simulink model "Exer2"  (R2014b)
settings: Solver=ode45  StartTime=0.0  StopTime=2  RelTol=1e-3
settings Model: Creator=Charlie  LastModifiedBy=Charlie

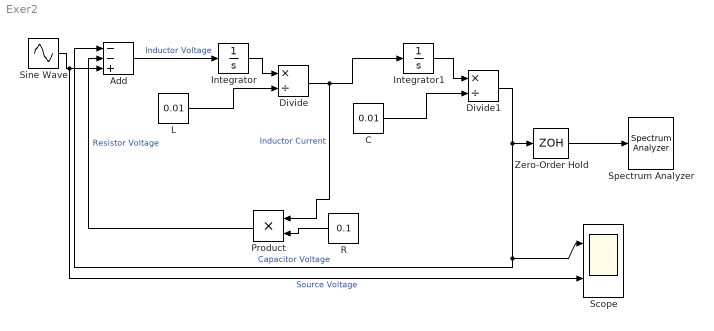
== system Exer2 ==
  Add : Sum  Inputs=--+
  C : Constant  Value=0.01
  Divide : Product  Inputs=*/
  Divide1 : Product  Inputs=*/
  Integrator : Integrator
  Integrator1 : Integrator
  L : Constant  Value=0.01
  Product : Product
  R : Constant  Value=0.1
  Scope : Scope  NumInputPorts=2
      settings: YMin=-2~-1  YMax=2~1
  Sine Wave : Sin  Frequency=20  SampleTime=0
  Spectrum Analyzer : SpectrumAnalyzer
  Zero-Order Hold : ZeroOrderHold  SampleTime=2e-5
  wires:
  Add/1 -> Integrator/1  "Inductor Voltage"
  Integrator/1 -> Divide/1
  L/1 -> Divide/2
  Divide/1 -> Product/1, Integrator1/1  "Inductor Current"
  Integrator1/1 -> Divide1/1
  C/1 -> Divide1/2
  Divide1/1 -> Zero-Order Hold/1, Scope/1, Add/1  "Capacitor Voltage"
  R/1 -> Product/2
  Product/1 -> Add/2  "Resistor Voltage"
  Zero-Order Hold/1 -> Spectrum Analyzer/1
  Sine Wave/1 -> Scope/2, Add/3  "Source Voltage"
